simulink model "SomanetTuning"  (R2016b)
settings: Solver=FixedStepDiscrete  StartTime=0.0  StopTime=inf  FixedStep=0.002  RelTol=1e-3  EnableMultiTasking=on
libraries: slrtlib x14, dspstat3 x2, xpcethercatlib x1
(part 2 of 2)

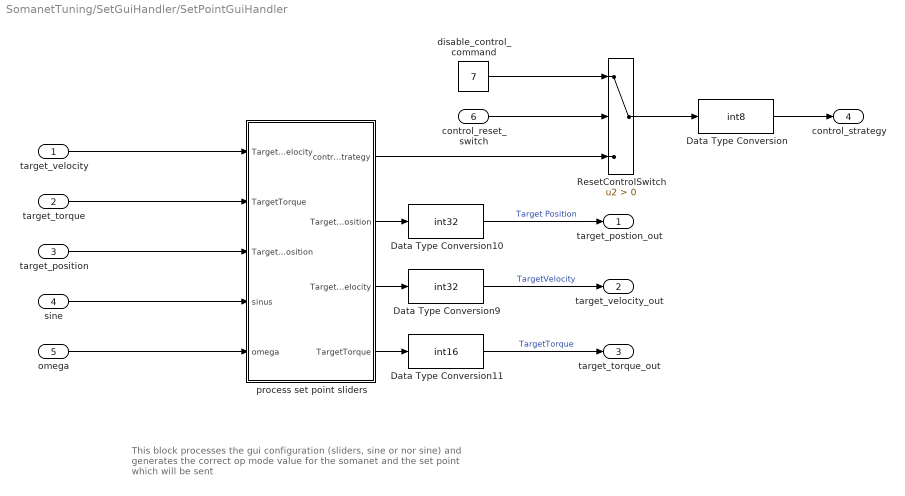
== system SomanetTuning/SetGuiHandler/SetPointGuiHandler ==
  note: This block processes the gui configuration (sliders, sine or nor sine)
      | and generates the correct op mode value for the somanet and the
      | set point which will be sent
  "target_velocity " : Inport
  target_torque : Inport  Port=2
  target_position : Inport  Port=3
  sine : Inport  Port=4
  omega : Inport  Port=5
  control_reset_switch : Inport  Port=6
  Data Type Conversion : DataTypeConversion  OutDataTypeStr=int8
  Data Type Conversion10 : DataTypeConversion  OutDataTypeStr=int32
  Data Type Conversion11 : DataTypeConversion  OutDataTypeStr=int16
  Data Type Conversion9 : DataTypeConversion  OutDataTypeStr=int32
  ResetControlSwitch : Switch  Criteria=u2 > Threshold
  disable_control_command : Constant  Value=7  OutDataTypeStr=int8
  process set point sliders : MATLAB Function  TreatAsAtomicUnit=on
  target_postion_out : Outport
  target_velocity_out : Outport  Port=2
  target_torque_out : Outport  Port=3
  control_strategy : Outport  Port=4
  wires:
  "target_velocity "/1 -> process set point sliders/1("TargetVelocity ")
  Data Type Conversion11/1 -> target_torque_out/1  "TargetTorque"
  process set point sliders/3(TargetVelocity) -> Data Type Conversion9/1
  sine/1 -> process set point sliders/4(sinus)
  process set point sliders/2(TargetPosition) -> Data Type Conversion10/1
  Data Type Conversion10/1 -> target_postion_out/1  "Target Position"
  omega/1 -> process set point sliders/5(omega)
  Data Type Conversion9/1 -> target_velocity_out/1  "TargetVelocity"
  target_position/1 -> process set point sliders/3("TargetPosition ")
  process set point sliders/4(TargetTorque) -> Data Type Conversion11/1
  target_torque/1 -> process set point sliders/2("TargetTorque ")
  control_reset_switch/1 -> ResetControlSwitch/2
  disable_control_command/1 -> ResetControlSwitch/1
  ResetControlSwitch/1 -> Data Type Conversion/1
  process set point sliders/1(control_strategy) -> ResetControlSwitch/3
  Data Type Conversion/1 -> control_strategy/1

== matlab function SomanetTuning/SetGuiHandler/SetPointGuiHandler/process set point sliders ==
  data: TargetVelocity input; control_strategy output; TargetTorque input; TargetPosition input; TargetPosition output; TargetVelocity output; TargetTorque output; sinus input; omega input
function [control_strategy, TargetPosition,TargetVelocity, TargetTorque] = fcn(TargetVelocity, TargetTorque, TargetPosition, sinus, omega)
    persistent last_V;
    persistent last_T;
    persistent last_P;
    persistent last_mode;
    stepsize = 0.1;
    
    if isempty(last_V)
        last_V = 0;
        last_T = 0;
        last_P = 0;
        last_mode = 0;
    end
    
    if sinus == 0
        omega = 1;
    end
     
    if or((sinus == 0),(sinus == 1))
        if TargetVelocity ~= last_V
            last_V = TargetVelocity;
            last_mode = 9;
            control_strategy = 9;
        elseif TargetTorque ~= last_T
            last_T = TargetTorque;
            last_mode = 10;
            control_strategy = 10;
        elseif TargetPosition ~= last_P
            last_P = TargetPosition;
            last_mode = 8;
            control_strategy = 8;
        else
            TargetPosition = omega*last_P;
            TargetVelocity = omega*last_V ;
            TargetTorque = omega*last_T ;
            control_strategy = last_mode;

        end
    else
        vStep = min(max(TargetVelocity - last_V, -stepsize), stepsize);
        tStep = min(max(TargetTorque - last_T, -stepsize), stepsize);
        pStep = min(max(TargetPosition - last_P, -stepsize), stepsize);
        TargetVelocity = last_V + vStep;
        TargetTorque = last_T + tStep;
        TargetPosition = last_P + pStep;
        if TargetVelocity ~= last_V
            last_V = TargetVelocity;
            last_mode = 9;
            control_strategy = 9;
        elseif TargetTorque ~= last_T
            last_T = TargetTorque;
            last_mode = 10;
            control_strategy = 10;
        elseif TargetPosition ~= last_P
            last_P = TargetPosition;
            last_mode = 8;
            control_strategy = 8;
        else
            control_strategy = last_mode;
        end
    end     
end

== matlab function SomanetTuning/MATLAB Function ==
  data: should_reinit output; state input; is_initializing output; is_updating output
function [should_reinit, is_initializing, is_updating] = enable_subsystems(state)
persistent reinit_timeout;
if(isempty(reinit_timeout))
    reinit_timeout = 0;
end
persistent is_initializing_pers;
persistent is_updating_pers;
persistent should_reinit_pers;
if isempty(is_initializing_pers)
    is_initializing_pers = false;
    is_updating_pers = false;
     should_reinit_pers = false;
end
switch state
    case State.startup
        should_reinit_pers = false;
        is_initializing_pers = true;
        is_updating_pers = false;
    case State.tuning
        should_reinit_pers = false;
        is_initializing_pers = false;
        is_updating_pers = true;
    case State.disconnected
        if(reinit_timeout == 0)
            should_reinit_pers = true;
            reinit_timeout = 500;
        else
            should_reinit_pers = false;
            reinit_timeout = reinit_timeout - 1;
        end
        is_initializing_pers = false;
        is_updating_pers = false;
    otherwise
        should_reinit_pers = false;
        is_initializing_pers = false;
        is_updating_pers = false;
end
    is_initializing = is_initializing_pers;
    is_updating = is_updating_pers;
    should_reinit = should_reinit_pers;

== stateflow chart SomanetTuning/Chart ==
  settings: stateMachineType=MOORE_MACHINE
  state somanet_connected
    state Initialize
      state startup_from_disconnect
        state = pending
        controlword = 128;
      state normal_startup
        state = pending
        op_mode_out = int8(0)
      state read_config
        state = startup
      state enter_tuning_mode
        op_mode_out = int8(-128)
      state exit_tuning_mode
        state = pending
        op_mode_out = int8(8)
      startup_from_disconnect -> enter_tuning_mode : [statusword==4160 | statusword==4176 | statusword==4192 | statusword== 4208]
      (default) -> startup_from_disconnect [order 1] : [statusword==4136 | statusword == 4104 | statusword == 4120 | statusword == 4152 | statusword == 4143]
      (default) -> normal_startup [order 2]
      normal_startup -> enter_tuning_mode : [statusword==0 | statusword==64 | statusword==4160 | statusword==4176 | statusword==4192 | statusword== 4208]
      enter_tuning_mode -> read_config : [op_mode_somanet == op_mode_out]
      read_config -> exit_tuning_mode : [ready_to_start == 1]
    state Operational
      state=sync
      state Switch_on_disabled
        state Choosing_control_mode
        state Sending_new_op_mode
          state Position_control
            op_mode_out = int8(8)
          state Tuning_mode
            op_mode_out = int8(-128)
          state Torque_control
            op_mode_out = int8(10)
          state Velocity_control
            op_mode_out = int8(9)
        state Request_to_switch_on
          controlword = 6
        (default) -> Choosing_control_mode
        Choosing_control_mode -> Position_control [order 1] : [op_mode_desired == 8]
        Choosing_control_mode -> Tuning_mode [order 4] : [op_mode_desired == -128]
        Choosing_control_mode -> Velocity_control [order 2] : [op_mode_desired == 9]
        Choosing_control_mode -> Torque_control [order 3] : [op_mode_desired ==10]
        Sending_new_op_mode -> Request_to_switch_on : [op_mode_out ~= -128 && op_mode_somanet == op_mode_out]
      state Ready_to_switch_on
        controlword = 7
      state Quick_stop_active_desired
        controlword = 2
      state Operation_enabled
      (default) -> Switch_on_disabled
      Request_to_switch_on -> Ready_to_switch_on : [(statusword==4129 | statusword == 4145 | statusword == 4160) && quick_stop_switch==0]
      Quick_stop_active_desired -> Switch_on_disabled : [statusword==4160 | statusword==4176 | statusword==4192 | statusword== 4208]
      Ready_to_switch_on -> Operation_enabled : [statusword==4135 | statusword == 4151]
      Operation_enabled -> Quick_stop_active_desired : [quick_stop_switch == 1 | op_mode_desired ~= op_mode_out]
    state TuningMode
      state Tuning
        state = tuning
      state Op_desired
        op_mode_out = int8(0)
      (default) -> Tuning
      Tuning -> Op_desired : [op_mode_desired ~= -128]
    state Fault
      state = fault
      state Fault
      state Fault_remove_desired
        controlword = 128;
      (default) -> somanet_connected.Fault.Fault
      somanet_connected.Fault.Fault -> Fault_remove_desired : [clear_fault_switch==1]
    (default) -> Initialize
    Operational -> somanet_connected.Fault [order 1] : [statusword==4136 | statusword == 4104 | statusword == 4120 | statusword == 4152 | statusword == 4143 | statusword == 4111]
    Operational -> TuningMode [order 2] : [op_mode_somanet == -128]
    TuningMode -> Operational : [op_mode_somanet ~= -128]
    exit_tuning_mode -> Operational : [op_mode_somanet == op_mode_out]
    Fault_remove_desired -> Operational : [statusword==4160 | statusword==4176 | statusword==4192 | statusword== 4208]
  state model_start
    state = pending
  state somanet_disconnected
    state = disconnected
  (default) -> model_start
  model_start -> somanet_connected : [errorcode~=0]
  somanet_disconnected -> somanet_connected : [errorcode~=0]
  somanet_connected -> somanet_disconnected : [errorcode==0]
  data: statusword input uint16; controlword output double; quick_stop_switch input boolean; clear_fault_switch input; op_mode_desired input int8; op_mode_somanet input; op_mode_out output int8; state output Enum: State; errorcode input; ready_to_start input

== matlab function SomanetTuning/determine_opmode/MATLAB Function ==
  data: control_strategy input; fixed_strategy output
function fixed_strategy = ignore_disable_control(control_strategy)
%% Ignores the 'disable control' command button
% When in tuning mode, one can send a disable control command, 7
% When the desired somanet state is cyclic synchronous, the opmode should
% stay the same when this button is accidentally pressed
% Therefore, the last valid strategy is returned
persistent last_strategy;
if(isempty(last_strategy)) 
    last_strategy = int8(0);
end
if(control_strategy ~= 7)
    fixed_strategy = control_strategy;
    last_strategy = control_strategy;
else
    fixed_strategy = last_strategy;
end

end
